simulink model "DC_model"  (R2024a)
settings: Solver=ode3  StartTime=Tstart  StopTime=Tstop  FixedStep=Tsim  RelTol=1e-3  EnableMultiTasking=on
values from neighbouring files (symbols this model uses):
  kth = 0    [DC_model_init.m]
  kw = 0    [DC_model_init.m]
  Ra = 0.075    [DC_model_init.m]
  Ta = 20e-3    (= 0.02)    [DC_model_init.m]
  Tm = 0.5    [DC_model_init.m]
  Tsim = 10e-3    (= 0.01)    [DC_model_init.m]
  Tth = 1    [DC_model_init.m]
  Ua = 1    [DC_model_init.m]
  Up = (1-Ra)    (= 0.925)    [DC_model_init.m]
settings Model: Creator=Pop  LastModifiedBy=lazar
settings SolverCC: AlgebraicLoopSolver=TrustRegion
settings DataIOCC: LimitDataPoints=on  SaveFormat=Array  ReturnWorkspaceOutputs=off
settings OptimizationCC: LifeSpan=inf
settings DebuggingCC: SolverPrmCheckMsg=warning  UnconnectedInputMsg=warning  UnconnectedOutputMsg=warning  UnconnectedLineMsg=warning  SFUnexpectedBacktrackingDiag=warning  SFNoUnconditionalDefaultTransitionDiag=warning  SFExecutionAtInitializationDiag=none  ArithmeticOperatorsInVariantConditions=warning
settings HardwareCC: ProdBitPerPointer=32  ProdBitPerSizeT=32  ProdBitPerPtrDiffT=32  ProdLargestAtomicFloat=None  ProdIntDivRoundTo=Undefined  ProdEndianess=Unspecified  ProdWordSize=32  ProdHWDeviceType=32-bit Generic
settings ModelReferenceCC: PropagateSignalLabelsOutOfModel=off
settings SFSimCC: SimUseLocalCustomCode=off  CustomCodeUndefinedFunction=UseInterfaceOnly
settings RTWCC: RTWUseLocalCustomCode=off  GPUComputeCapability=3.5
settings CodeAppCC: StateflowObjectComments=on
settings GRTTargetCC: TargetLangStandard=C89/C90 (ANSI)
settings ConfigComp: CovMetricSettings=dw  CovSaveCumulativeToWorkspaceVar=on  CovSaveSingleToWorkspaceVar=on  CovExternalEMLEnable=off  CovSFcnEnable=off

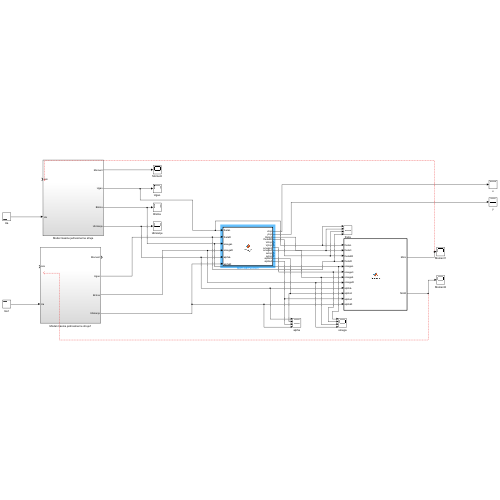
[thumbnail: Simulink's stored preview of the top-level diagram]
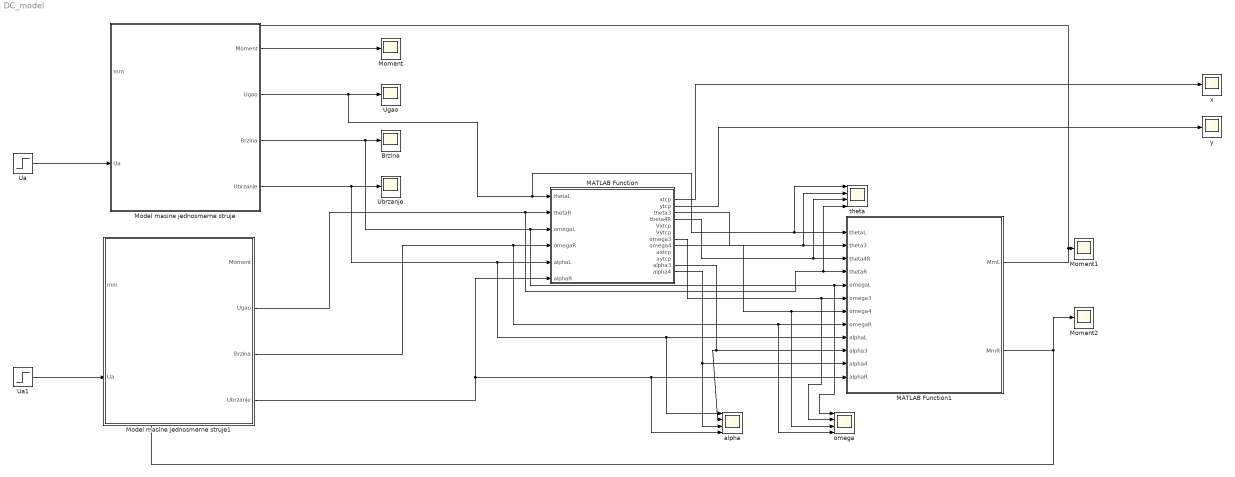
== system DC_model ==
  Brzina : Scope
  MATLAB Function : MATLAB Function  TreatAsAtomicUnit=on
  MATLAB Function1 : MATLAB Function  TreatAsAtomicUnit=on
  Model masine jednosmerne struje : Subsystem
  Model masine jednosmerne struje1 : Subsystem
  Moment : Scope
  Moment1 : Scope
  Moment2 : Scope
  Ua : Step  Time=0  After=Ua  SampleTime=Tsim
  Ua1 : Step  Time=0  After=-Ua/4  SampleTime=Tsim
  Ubrzanje : Scope
  Ugao : Scope
  alpha : Scope  NumInputPorts=4
  omega : Scope  NumInputPorts=4
  theta : Scope  NumInputPorts=4
  x : Scope
  y : Scope
  wires:
  Model masine jednosmerne struje/3(Brzina) -> omega/1, MATLAB Function1/5(omegaL), MATLAB Function/3(omegaL), Brzina/1
  Model masine jednosmerne struje/1(Moment) -> Moment/1
  Ua/1 -> Model masine jednosmerne struje/2(Ua)
  Model masine jednosmerne struje/4(Ubrzanje) -> alpha/1, MATLAB Function1/9(alphaL), MATLAB Function/5(alphaL), Ubrzanje/1
  Ua1/1 -> Model masine jednosmerne struje1/2(Ua)
  Model masine jednosmerne struje1/2(Ugao) -> theta/4, MATLAB Function1/4(thetaR), MATLAB Function/2(thetaR)
  Model masine jednosmerne struje1/4(Ubrzanje) -> MATLAB Function/6(alphaR), alpha/4, MATLAB Function1/12(alphaR)
  MATLAB Function/1(xtcp) -> x/1
  MATLAB Function/2(ytcp) -> y/1
  MATLAB Function/3(theta3) -> theta/2, MATLAB Function1/2(theta3)
  MATLAB Function/4(theta4R) -> theta/3, MATLAB Function1/3(theta4R)
  MATLAB Function/7(omega3) -> omega/2, MATLAB Function1/6(omega3)
  MATLAB Function/8(omega4) -> omega/3, MATLAB Function1/7(omega4)
  MATLAB Function/11(alpha3) -> MATLAB Function1/10(alpha3), alpha/2
  MATLAB Function/12(alpha4) -> alpha/3, MATLAB Function1/11(alpha4)
  MATLAB Function1/1(MmL) -> Moment1/1
  MATLAB Function1/2(MmR) -> Moment2/1
  Model masine jednosmerne struje/2(Ugao) -> theta/1, MATLAB Function1/1(thetaL), MATLAB Function/1(thetaL), Ugao/1
  Model masine jednosmerne struje1/3(Brzina) -> omega/4, MATLAB Function1/8(omegaR), MATLAB Function/4(omegaR)

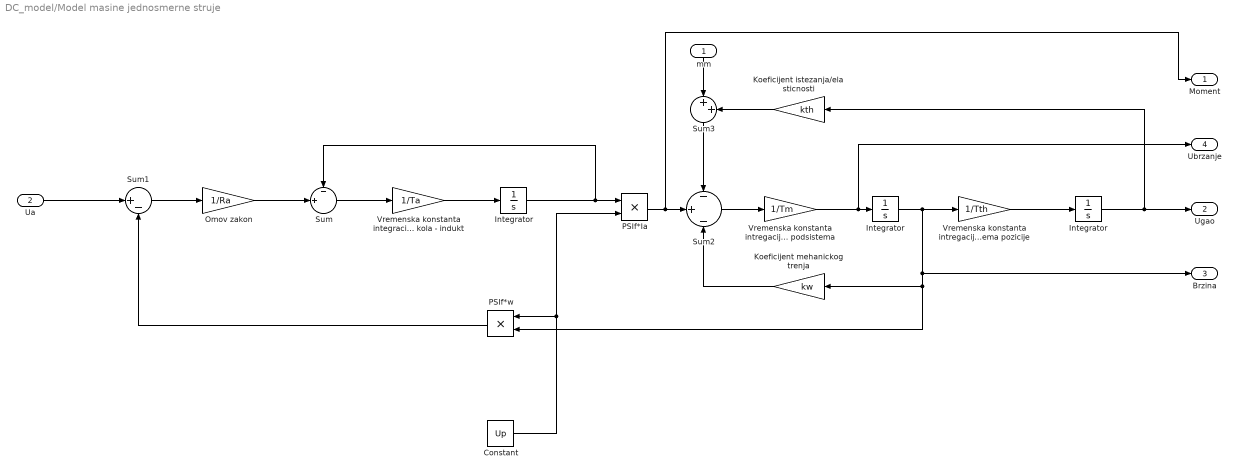
== system DC_model/Model masine jednosmerne struje ==
  mm : Inport
  Ua : Inport  Port=2
  "   Integrator   " : Integrator
  "  Integrator  " : Integrator
  Constant : Constant  Value=Up
  Integrator : Integrator
  Koeficijent istezanja/elasticnosti : Gain  Gain=kth  SampleTime=Tsim
  Koeficijent mehanickog trenja : Gain  Gain=kw  SampleTime=Tsim
  Omov zakon : Gain  Gain=1/Ra  SampleTime=Tsim
  PSIf*Ia : Product  SampleTime=Tsim
  PSIf*w : Product  SampleTime=Tsim
  Sum : Sum  Inputs=-|+||  SampleTime=Tsim
  Sum1 : Sum  Inputs=|+-  SampleTime=Tsim
  Sum2 : Sum  Inputs=-||+||-  SampleTime=Tsim
  Sum3 : Sum  Inputs=|++  SampleTime=Tsim
  Vremenska konstanta integracije rotorskog kola - indukt : Gain  Gain=1/Ta  SampleTime=Tsim
  Vremenska konstanta intregacije mehanickog podsistema : Gain  Gain=1/Tm  SampleTime=Tsim
  Vremenska konstanta intregacije podsistema pozicije : Gain  Gain=1/Tth  SampleTime=Tsim
  Moment : Outport
  Ugao : Outport  Port=2
  Brzina : Outport  Port=3
  Ubrzanje : Outport  Port=4
  wires:
  Omov zakon/1 -> Sum/2
  Sum1/1 -> Omov zakon/1
  Integrator/1 -> Sum/1, PSIf*Ia/1
  Sum/1 -> Vremenska konstanta integracije rotorskog kola - indukt/1
  Vremenska konstanta integracije rotorskog kola - indukt/1 -> Integrator/1
  PSIf*Ia/1 -> Moment/1, Sum2/2
  Sum2/1 -> Vremenska konstanta intregacije mehanickog podsistema/1
  Vremenska konstanta intregacije mehanickog podsistema/1 -> Ubrzanje/1, "  Integrator  "/1
  Koeficijent mehanickog trenja/1 -> Sum2/3
  Vremenska konstanta intregacije podsistema pozicije/1 -> "   Integrator   "/1
  Sum3/1 -> Sum2/1
  Koeficijent istezanja/elasticnosti/1 -> Sum3/2
  Constant/1 -> PSIf*w/1, PSIf*Ia/2
  PSIf*w/1 -> Sum1/2
  "   Integrator   "/1 -> Koeficijent istezanja/elasticnosti/1, Ugao/1
  "  Integrator  "/1 -> Vremenska konstanta intregacije podsistema pozicije/1, PSIf*w/2, Koeficijent mehanickog trenja/1, Brzina/1
  Ua/1 -> Sum1/1
  mm/1 -> Sum3/1

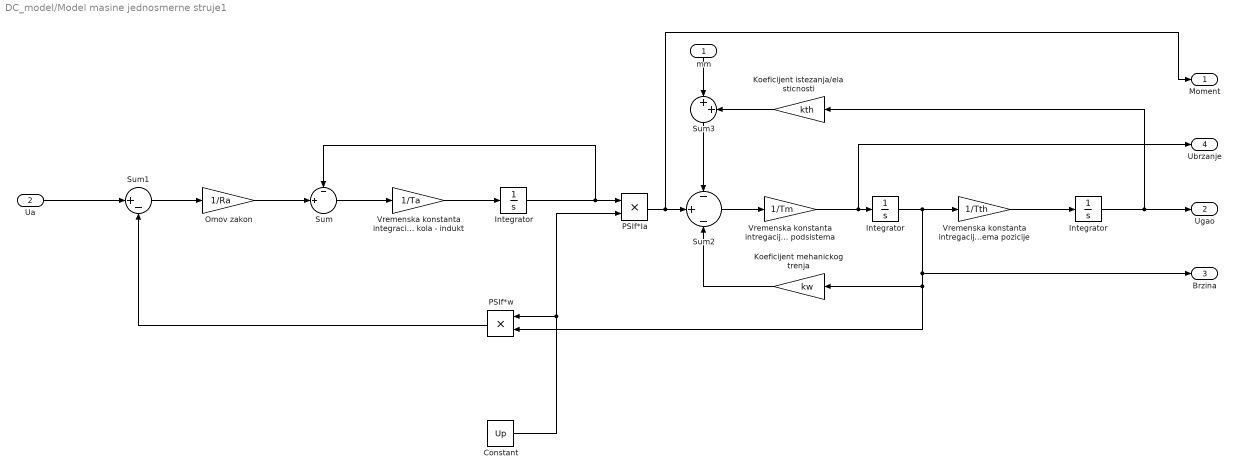
== system DC_model/Model masine jednosmerne struje1 ==
  mm : Inport
  Ua : Inport  Port=2
  "   Integrator   " : Integrator
  "  Integrator  " : Integrator
  Constant : Constant  Value=Up
  Integrator : Integrator
  Koeficijent istezanja/elasticnosti : Gain  Gain=kth  SampleTime=Tsim
  Koeficijent mehanickog trenja : Gain  Gain=kw  SampleTime=Tsim
  Omov zakon : Gain  Gain=1/Ra  SampleTime=Tsim
  PSIf*Ia : Product  SampleTime=Tsim
  PSIf*w : Product  SampleTime=Tsim
  Sum : Sum  Inputs=-|+||  SampleTime=Tsim
  Sum1 : Sum  Inputs=|+-  SampleTime=Tsim
  Sum2 : Sum  Inputs=-||+||-  SampleTime=Tsim
  Sum3 : Sum  Inputs=|++  SampleTime=Tsim
  Vremenska konstanta integracije rotorskog kola - indukt : Gain  Gain=1/Ta  SampleTime=Tsim
  Vremenska konstanta intregacije mehanickog podsistema : Gain  Gain=1/Tm  SampleTime=Tsim
  Vremenska konstanta intregacije podsistema pozicije : Gain  Gain=1/Tth  SampleTime=Tsim
  Moment : Outport
  Ugao : Outport  Port=2
  Brzina : Outport  Port=3
  Ubrzanje : Outport  Port=4
  wires:
  Omov zakon/1 -> Sum/2
  Sum1/1 -> Omov zakon/1
  Integrator/1 -> Sum/1, PSIf*Ia/1
  Sum/1 -> Vremenska konstanta integracije rotorskog kola - indukt/1
  Vremenska konstanta integracije rotorskog kola - indukt/1 -> Integrator/1
  PSIf*Ia/1 -> Moment/1, Sum2/2
  Sum2/1 -> Vremenska konstanta intregacije mehanickog podsistema/1
  Vremenska konstanta intregacije mehanickog podsistema/1 -> Ubrzanje/1, "  Integrator  "/1
  Koeficijent mehanickog trenja/1 -> Sum2/3
  Vremenska konstanta intregacije podsistema pozicije/1 -> "   Integrator   "/1
  Sum3/1 -> Sum2/1
  Koeficijent istezanja/elasticnosti/1 -> Sum3/2
  Constant/1 -> PSIf*w/1, PSIf*Ia/2
  PSIf*w/1 -> Sum1/2
  "   Integrator   "/1 -> Koeficijent istezanja/elasticnosti/1, Ugao/1
  "  Integrator  "/1 -> Vremenska konstanta intregacije podsistema pozicije/1, PSIf*w/2, Koeficijent mehanickog trenja/1, Brzina/1
  Ua/1 -> Sum1/1
  mm/1 -> Sum3/1

== matlab function DC_model/MATLAB Function1 ==
  data: thetaL input; MmL output; theta3 input; theta4R input; thetaR input; omegaL input; omega3 input; omega4 input; omegaR input; alphaL input; alpha3 input; alpha4 input; alphaR input; MmR output
function [MmL, MmR] = dinamics(thetaL, theta3, theta4R, thetaR, omegaL, omega3, omega4, omegaR, alphaL, alpha3, alpha4, alphaR)
    % Get parameters
    [~, P, D, mP, mD, JsP, JsD] = get_params();
    
    % Mass and moments of inertia
    m2 = mP; m3 = mD; m4 = mD; m5 = mP;
    Js2 = JsP; Js3 = JsD; Js4 = JsD; Js5 = JsP;
    
    % Accelerations of each mass center
    as2x = - P/2 * omegaL^2 * cos(thetaL) - P/2 * alphaL * sin(thetaL);
    as2y = - P/2 * omegaL^2 * sin(thetaL) + P/2 * alphaL * cos(thetaL);
    as3x = - P * omegaL^2 * cos(thetaL) - P * alphaL * sin(thetaL) - D/2 * omega3^2 * cos(theta3) - D/2 * alpha3 * sin(theta3);
    as3y = - P * omegaL^2 * sin(thetaL) + P * alphaL * cos(thetaL) - D/2 * omega3^2 * sin(theta3) + D/2 * alpha3 * cos(theta3);
    as4x = - P * omegaR^2 * cos(thetaR) - P * alphaR * sin(thetaR) - D/2 * omega4^2 * cos(theta4R) - D/2 * alpha4 * sin(theta4R);
    as4y = - P * omegaR^2 * sin(thetaR) + P * alphaR * cos(thetaR) - D/2 * omega4^2 * sin(theta4R) + D/2 * alpha4 * cos(theta4R);
    as5x = - P/2 * omegaR^2 * cos(thetaR) - P/2 * alphaR * sin(thetaR);
    as5y = - P/2 * omegaR^2 * sin(thetaR) + P/2 * alphaR * cos(thetaR);

    % Coefficient matrices
    A = [
        0, 0, -P/2*sin(thetaL), 0, 0, 0, 0, 0, 0, 0, 0, 0;
        0, 0, P/2*cos(thetaL), 0, 0, 0, 0, 0, 0, 0, 0, 0;
        -1, 0, 0, 0, 0, 0, -1, 0, 0, 0, 0, 0;
        0, 0, -D/2*sin(theta3), 0, 0, 0, 0, -D/2*sin(theta3), 0, 0, 0, 0;
        0, 0, D/2*cos(theta3), 0, 0, 0, 0, D/2*cos(theta3), 0, 0, 0, 0;
        0, -1, 0, 0, 0, 0, 0, 0, 0, 0, 0, 0;
        0, 0, 0, -1, 0, 0, 0, 0, 0, -1, 0, 0;
        0, 0, 0, 0, -D/2*sin(theta4R), 0, 0, 0, -D/2*sin(theta4R), 0, 0, 0;
        0, 0, 0, 0, D/2*cos(theta4R), 0, 0, 0, D/2*cos(theta4R), 0, 0, 0;
        0, 0, 0, 0, 0, -1, 0, 0, 0, 0, -1, 0;
        0, 0, 0, 0, 0, 0, 0, 0, 0, -P/2*sin(thetaR), 0, 0;
        0, 0, 0, 0, 0, 0, 0, 0, 0, P/2*cos(thetaR), 0, 0;
    ];

    b = [
        m2 * as2x; 
        m2 * as2y;
        Js2 * alphaL;
        m3 * as3x;
        m3 * as3y;
        Js3 * alpha3;
        m4 * as4x;
        m4 * as4y;
        Js4 * alpha4;
        m5 * as5x;
        m5 * as5y;
        Js5 * alphaR;
    ];

    % Solve the system
    solution = A\b;
    
    % Extract results
    ML = solution(3); 
    MR = solution(12); 
    
    MmL = ML;
    MmR = MR;
end

== matlab function DC_model/MATLAB Function ==
  data: thetaL input; xtcp output; thetaR input; omegaL input; omegaR input; alphaL input; alphaR input; ytcp output; theta3 output; theta4R output; Vxtcp output; Vytcp output; omega3 output; omega4 output; axtcp output; aytcp output; alpha3 output; alpha4 output
function [xtcp, ytcp, theta3, theta4R, Vxtcp, Vytcp, omega3, omega4, axtcp, aytcp, alpha3, alpha4] = forw_k(thetaL, thetaR, omegaL, omegaR, alphaL, alphaR)
    [L,P,D] = get_params();

    xA = -L/2 + P * cos(thetaL);
    yA = P * sin(thetaL);
    xB = L/2 + P * cos(thetaR);
    yB = P * sin(thetaR);

    A = (xB - xA) / D;
    B = (yB - yA) / D;
    C = (A*A + B*B) / 2;

    theta4R = 2*atan2(-B-sqrt(A*A+B*B-C*C), C-A);
    theta3 = asin((yB-yA)/D + sin(theta4R));
    xtcp = xA + D*cos(theta3);
    ytcp = yA + D*sin(theta3);

    % Velocities
    A_v = [ -1/(P*sin(thetaL)), 0, - D*sin(theta3)/(P*sin(thetaL)), 0;
            -1/(P*sin(thetaR)), 0, - D*sin(theta4R)/(P*sin(thetaR)), 0;
            0, 1/(P*cos(thetaL)), - D*cos(theta3)/(P*cos(thetaL)), 0;
            0, 1/(P*cos(thetaR)), 0, - D*cos(theta4R)/(P*cos(thetaR))
            ];
    B_v = [   omegaL;
            omegaR;
            omegaL;
            omegaR
            ];
    V = A_v\B_v;
    Vxtcp = V(1);
    Vytcp = V(2);
    omega3 = V(3);
    omega4 = V(4);

    % Accelerations
    A_a = [-P*sin(thetaL), 0, -D*sin(theta3), 0;
           0, -P*sin(thetaR), 0, -D*sin(theta4R);
           P*cos(thetaL), 0, D*cos(theta3), 0;
           0, P*cos(thetaR), 0, D*cos(theta4R)];

    b_a = [- P*cos(thetaL)*omegaL^2 - P*sin(thetaL)*alphaL - D*cos(theta3)*omega3^2;
            - P*cos(thetaR)*omegaR^2 - P*sin(thetaR)*alphaR - D*cos(theta4R)*omega4^2;
            - P*sin(thetaL)*omegaL^2 + P*cos(thetaL)*alphaL - D*sin(theta3)*omega3^2;
            - P*sin(thetaR)*omegaR^2 + P*cos(thetaR)*alphaR - D*sin(theta4R)*omega4^2];

    a = A_a\b_a;
    axtcp = a(1);
    aytcp = a(2);
    alpha3 = a(3);
    alpha4 = a(4);
end
